simulink model "PubIfDecisionLM_MDL"  (R2020b)
settings: configuration reference "DspaceConfig" (kept outside this file)
PostLoadFcn:
  | if any(exist('dsrtsu_mdlpostloadfcn', 'file') ~= 0), dsrtsu_mdlpostloadfcn('Execute', bdroot); end
InitFcn:
  | , if any(exist('dsmpb_private', 'file') ~= 0), dsmpb_private('dsmpb_mdlclblib', 'Init', bdroot); end,
undefined symbols (not defined in the file or in its folder): OFM_OBJ_FUSIONTYPE_E, OFM_OBJ_MOVINGSTATE_E, OFM_OBJ_ORIENTATION_E, OFM_OBJ_TYPE_E, P_LM_Cyc, P_LM_EMLHistKapRcdBufSize, P_LM_EMLHistTrajBaseDis, P_LM_EMLHistTrajPNum, P_LM_EMLKapCorrMaxThre, P_LM_EMLMinKapThre, P_LM_EMLPathDisDiffThre, P_LM_EMLQuaFiltPar, P_LM_EMLTurnActKapThre, P_LM_EMLValidQuaThre, P_LM_FntPath1Disgap, P_LM_FntPath1MinDis, P_LM_FntPath1Timegap, P_LM_FntPath2Disgap, P_LM_FntPath2MinDis, P_LM_FntPath2Timegap, P_LM_FntPath3Disgap, P_LM_FntPath3MinDis, P_LM_FntPath3Timegap, P_LM_FusBLParFiltP, P_LM_FusEVDifC2Thre, P_LM_FusEVOPath1AllVSLDisThre, P_LM_FusEVOPath1AllVSLLostNumThre, P_LM_FusEVOPath1AllVSLQuaThre, P_LM_FusEVOPath1OTLFacNLC, P_LM_FusOTLQuaThre, P_LM_FusOTLSW, P_LM_FusParC0Index, P_LM_FusParC1Index, P_LM_FusParC2Index, P_LM_FusParC3Index, P_LM_FusVSLQuaThre, P_LM_FusVSLSW, P_LM_FusVSLValidSteerWheerAngThre, P_LM_FusVSLValidVxvThre, P_LM_LaneWidth, P_LM_OTLBufTPInfoEvaFactor, P_LM_OTLObjNum, P_LM_OTLObjSelectAgeThre, P_LM_OTLObjSelectDxAssessVx, P_LM_OTLObjSelectDxThre, P_LM_OTLObjSelectVxThre, P_LM_OTLObjSelectVyAssessDx, P_LM_OTLObjSelectVyThre, P_LM_OTLTrajPntBaseDis, P_LM_OTLTrajStdThre, P_LM_VSLAvailLineNum, P_LM_VSLBLSDiffThre, P_LM_VSLBLSDisRatio, P_LM_VSLFusBLParFiltP_C1, P_LM_VSLFusBLParFiltP_C2, P_LM_VSLFusBLParFiltP_C3, P_LM_VSLFusBLParFiltP_Quality, P_LM_VSLHistTrajBaseDis, P_LM_VSLHistTrajPNum, P_LM_VSLLCC0diff ... (+18)
libraries: simulink x145, LM_LIB x43
(part 2 of 24)

== system PubIfDecisionLM_MDL/Subsystem2/LM_EML/LM_EMLRearPath1 ==
  VxvRef_ms : Inport
  LM_ComEVOffsetX : Inport  Port=2
  LM_ComEVOffsetY : Inport  Port=3
  LM_ComEVOffsetAng : Inport  Port=4
  LM_RearPath1Dis : Inport  Port=5
  LM_RearPath2Dis : Inport  Port=6
  LM_RearPath3Dis : Inport  Port=7
  VehStandstill : Inport  Port=8
  LM_EMLEgoTrajRecorddFlgCalc : Subsystem
  LM_EMLHistTrajCoordinateConvert : Subsystem
  LM_EMLHistTrajRecordBufferInfo : Subsystem
  LM_EMLHistTrajRecordBufferUpdate : Subsystem
  MATLAB Function : MATLAB Function  TreatAsAtomicUnit=on
  Unit Delay1 : UnitDelay  InitialCondition=zeros(80,1)  SampleTime=-1  HasFrameUpgradeWarning=on
  Unit Delay4 : UnitDelay  InitialCondition=zeros(80,1)  SampleTime=-1  HasFrameUpgradeWarning=on
  LM_EMLRearPath1P : Outport
  LM_EMLRearPath1Qulity : Outport  Port=2
  LM_EMLRearPath2P : Outport  Port=3
  LM_EMLRearPath2Qulity : Outport  Port=4
  LM_EMLRearPath3P : Outport  Port=5
  LM_EMLRearPath3Qulity : Outport  Port=6
  wires:
  LM_EMLEgoTrajRecorddFlgCalc/1(LM_EMLHistTrajRcdFlg) -> LM_EMLHistTrajRecordBufferUpdate/3(LM_EMLHistTrajRcdFlg), LM_EMLHistTrajRecordBufferInfo/1(LM_EMLHistTrajRcdFlg)
  LM_EMLHistTrajRecordBufferInfo/1(LM_EMLHistPEndPos) -> LM_EMLHistTrajRecordBufferUpdate/4(LM_EMLHistPEndPos), MATLAB Function/3(LM_EMLHistPEndPos)
  LM_EMLHistTrajCoordinateConvert/1(LM_EMLHistTrajVectXK1Adju) -> LM_EMLHistTrajRecordBufferUpdate/1(LM_EMLHistTrajVectXK1Adju)
  LM_EMLHistTrajRecordBufferUpdate/2(LM_EMLHistTrajVectY) -> Unit Delay4/1, MATLAB Function/2(LM_EMLHistTrajVectY)
  VehStandstill/1 -> LM_EMLEgoTrajRecorddFlgCalc/1(VehStandstill), LM_EMLHistTrajCoordinateConvert/6(VehStandstill)
  LM_ComEVOffsetX/1 -> LM_EMLHistTrajCoordinateConvert/3(LM_ComEVOffsetX)
  LM_ComEVOffsetY/1 -> LM_EMLHistTrajCoordinateConvert/4(LM_ComEVOffsetY)
  VxvRef_ms/1 -> LM_EMLEgoTrajRecorddFlgCalc/2(VxvRef_ms)
  LM_EMLHistTrajCoordinateConvert/2(LM_EMLHistTrajVectYK1Adju) -> LM_EMLHistTrajRecordBufferUpdate/2(LM_EMLHistTrajVectYK1Adju)
  LM_ComEVOffsetAng/1 -> LM_EMLHistTrajCoordinateConvert/5(LM_ComEVOffsetAng)
  LM_EMLHistTrajRecordBufferUpdate/1(LM_EMLHistTrajVectX) -> Unit Delay1/1, MATLAB Function/1(LM_EMLHistTrajVectX)
  LM_EMLHistTrajRecordBufferInfo/2(LM_EMLHistPFristPos) -> MATLAB Function/4(LM_EMLHistPFristPos)
  LM_EMLHistTrajRecordBufferInfo/3(LM_EMLHistPNum) -> MATLAB Function/5(LM_EMLHistPNum)
  MATLAB Function/1(LM_EMLRearPath1P) -> LM_EMLRearPath1P/1  "LM_EMLRearPath1P"
  MATLAB Function/2(LM_EMLRearPath1Qulity) -> LM_EMLRearPath1Qulity/1  "LM_EMLRearPath1Qulity"
  MATLAB Function/6(LM_EMLRearPath3Qulity) -> LM_EMLRearPath3Qulity/1  "LM_EMLRearPath3Qulity"
  MATLAB Function/3(LM_EMLRearPath2P) -> LM_EMLRearPath2P/1  "LM_EMLRearPath2P"
  MATLAB Function/4(LM_EMLRearPath2Qulity) -> LM_EMLRearPath2Qulity/1  "LM_EMLRearPath2Qulity"
  MATLAB Function/5(LM_EMLRearPath3P) -> LM_EMLRearPath3P/1  "LM_EMLRearPath3P"
  Unit Delay1/1 -> LM_EMLHistTrajCoordinateConvert/1(LM_EMLHistTrajVectXK1)
  Unit Delay4/1 -> LM_EMLHistTrajCoordinateConvert/2(LM_EMLHistTrajVectYK1)
  LM_RearPath1Dis/1 -> MATLAB Function/6(LM_RearPath1Dis)
  LM_RearPath2Dis/1 -> MATLAB Function/7(LM_RearPath2Dis)
  LM_RearPath3Dis/1 -> MATLAB Function/8(LM_RearPath3Dis)

== system PubIfDecisionLM_MDL/Subsystem2/LM_Fusion1/LM_FusBaseLineFilt ==
  DIR_BUS : Inport
  LM_C0Info : Inport  Port=2
  LM_FusBLInfo : Inport  Port=3
  Bus Creator : BusCreator  Inputs=4  OutDataTypeStr=Bus: LM_FusC0InfoBus  NonVirtualBus=on
  Bus Creator1 : BusCreator  Inputs=6  OutDataTypeStr=Bus: LM_FusBLInfoBus  NonVirtualBus=on
  Bus Selector : BusSelector  OutputSignals=LM_LLC0,LM_LRC0,LM_RLC0,LM_RRC0
  Bus Selector1 : BusSelector  OutputSignals=DIR_LC2LeValid,DIR_LC2RigValid
  LM_FusBaseLineC0Filt : Subsystem
  LM_FusBaseLineInfoFilt : Subsystem
  Subsystem1 : Subsystem  Commented=on
  LM_FusBLInfoFilt : Outport
  LM_C0InfoFilt : Outport  Port=2
  wires:
  LM_C0Info/1 -> Bus Selector/1
  DIR_BUS/1 -> Bus Selector1/1
  Bus Selector1/1 -> LM_FusBaseLineC0Filt/1(DIR_LC2LeValid)  "<DIR_LC2LeValid>"
  Bus Selector1/2 -> LM_FusBaseLineC0Filt/2(DIR_LC2RigValid)  "<DIR_LC2RigValid>"
  Bus Selector/1 -> LM_FusBaseLineC0Filt/3(LM_LLC0BefFilt)  "<LM_LLC0>"
  Bus Selector/2 -> LM_FusBaseLineC0Filt/4(LM_LRC0BefFilt)  "<LM_LRC0>"
  Bus Selector/3 -> LM_FusBaseLineC0Filt/5(LM_RLC0BefFilt)  "<LM_RLC0>"
  Bus Selector/4 -> LM_FusBaseLineC0Filt/6(LM_RRC0BefFilt)  "<LM_RRC0>"
  LM_FusBaseLineC0Filt/1(LM_LLC0) -> Bus Creator/1
  LM_FusBaseLineC0Filt/2(LM_LRC0) -> Bus Creator/2
  LM_FusBaseLineC0Filt/3(LM_RLC0) -> Bus Creator/3
  LM_FusBaseLineC0Filt/4(LM_RRC0) -> Bus Creator/4
  Bus Creator/1 -> LM_C0InfoFilt/1  "LM_C0InfoFilt"
  LM_FusBaseLineInfoFilt/1(LM_FusBLFntPath1Info) -> Bus Creator1/1
  LM_FusBaseLineInfoFilt/2(LM_FusBLFntPath2Info) -> Bus Creator1/2
  LM_FusBaseLineInfoFilt/3(LM_FusBLFntPath3Info) -> Bus Creator1/3
  LM_FusBaseLineInfoFilt/4(LM_FusBLRearPath1Info) -> Bus Creator1/4
  LM_FusBaseLineInfoFilt/5(LM_FusBLRearPath2Info) -> Bus Creator1/5
  LM_FusBaseLineInfoFilt/6(LM_FusBLRearPath3Info) -> Bus Creator1/6
  LM_FusBLInfo/1 -> LM_FusBaseLineInfoFilt/1(LM_FusBLInfo)
  Bus Creator1/1 -> LM_FusBLInfoFilt/1  "LM_FusBLInfoFilt"

== system PubIfDecisionLM_MDL/Subsystem2/LM_Fusion1/LM_FusBaseLineInfoCalc ==
  LM_FusBLInfo : Inport
  LM_VSL : Inport  Port=2
  LM_EML : Inport  Port=3
  LM_OTL : Inport  Port=4
  LM_REL : Inport  Port=5
  LM_MAL : Inport  Port=6
  Bus Selector : BusSelector  OutputSignals=LM_FusFntPathK
  LM_FusBLFntPath1 : Subsystem  Commented=on
  LM_FusBLFntPath1130 : Subsystem  Commented=on
  LM_FusBLFntPath2 : Subsystem  Commented=on
  LM_FusBLFntPath3 : Subsystem
  LM_FusBLRearPath : Subsystem
  LM_FusBLFntPath1Info : Outport
  LM_FusBLFntPath2Info : Outport  Port=2
  LM_FusBLFntPath3Info : Outport  Port=3
  LM_FusBLRearPath1Info : Outport  Port=4
  LM_FusBLRearPath2Info : Outport  Port=5
  LM_FusBLRearPath3Info : Outport  Port=6
  wires:
  LM_FusBLInfo/1 -> Bus Selector/1
  LM_FusBLRearPath/1(LM_FusBLRearPath1Info) -> LM_FusBLRearPath1Info/1
  LM_FusBLRearPath/2(LM_FusBLRearPath2Info) -> LM_FusBLRearPath2Info/1
  LM_FusBLRearPath/3(LM_FusBLRearPath3Info) -> LM_FusBLRearPath3Info/1
  LM_EML/1 -> LM_FusBLFntPath3/1(LM_EML)
  LM_VSL/1 -> LM_FusBLRearPath/1(LM_VSL), LM_FusBLFntPath3/2(LM_VSL)
  LM_OTL/1 -> LM_FusBLFntPath3/3(LM_OTL)
  Bus Selector/1 -> LM_FusBLFntPath3/6(LM_FusFntPathK)  "<LM_FusFntPathK>"
  LM_REL/1 -> LM_FusBLFntPath3/4(LM_REL)
  LM_MAL/1 -> LM_FusBLFntPath3/5(LM_MAL)
  LM_FusBLFntPath3/1(LM_FusBLFntPath1Info) -> LM_FusBLFntPath1Info/1
  LM_FusBLFntPath3/2(LM_FusBLFntPath2Info) -> LM_FusBLFntPath2Info/1
  LM_FusBLFntPath3/3(LM_FusBLFntPath3Info) -> LM_FusBLFntPath3Info/1

== system PubIfDecisionLM_MDL/Subsystem2/LM_Fusion1/LM_FusLaneModelInfo ==
  LM_FusBLInfoFilt : Inport
  LM_C0InfoFilt : Inport  Port=2
  LM_ComBus : Inport  Port=3
  LM_FusfCamValidInfo : Inport  Port=4
  Bus Selector : BusSelector  OutputSignals=LM_LLC0
  Bus Selector1 : BusSelector  OutputSignals=LM_PathDisBus
  Bus Selector2 : BusSelector  OutputSignals=LM_LRC0
  Bus Selector3 : BusSelector  OutputSignals=LM_RLC0
  Bus Selector4 : BusSelector  OutputSignals=LM_RRC0
  LM_LLInfo : LM_LIB/LM_LineInfo1  SystemSampleTime=-1  VariantActivationTime=update diagram  Latency=0  AutoFrameSizeCalculation=off
  LM_LRInfo : LM_LIB/LM_LineInfo1  SystemSampleTime=-1  VariantActivationTime=update diagram  Latency=0  AutoFrameSizeCalculation=off
      link override LM_Line_Fnt/LM_Path04/Constant1: Value=1
  LM_RLInfo : LM_LIB/LM_LineInfo1  SystemSampleTime=-1  VariantActivationTime=update diagram  Latency=0  AutoFrameSizeCalculation=off
  LM_RRInfo : LM_LIB/LM_LineInfo1  SystemSampleTime=-1  VariantActivationTime=update diagram  Latency=0  AutoFrameSizeCalculation=off
  Signal Conversion{,1..7} (8 alike) : SignalConversion  OverrideOpt=off
  LM_LINE_LL : Outport  BusOutputAsStruct=on
  LM_LINE_LR : Outport  Port=2  BusOutputAsStruct=on
  LM_LINE_RL : Outport  Port=3  BusOutputAsStruct=on
  LM_LINE_RR : Outport  Port=4  BusOutputAsStruct=on
  wires:
  LM_C0InfoFilt/1 -> Bus Selector4/1, Bus Selector3/1, Bus Selector2/1, Bus Selector/1
  Bus Selector1/1 -> LM_LLInfo/3, LM_RRInfo/3, LM_RLInfo/3, LM_LRInfo/3  "<LM_PathDisBus>"
  LM_FusBLInfoFilt/1 -> LM_LLInfo/1, LM_RRInfo/1, LM_RLInfo/1, LM_LRInfo/1
  Bus Selector/1 -> Signal Conversion2/1  "<LM_LLC0>"
  Bus Selector2/1 -> Signal Conversion1/1  "<LM_LRC0>"
  Bus Selector3/1 -> Signal Conversion/1  "<LM_RLC0>"
  Signal Conversion/1 -> LM_RLInfo/2  "LM_LineC0"
  Signal Conversion1/1 -> LM_LRInfo/2  "LM_LineC0"
  Signal Conversion2/1 -> LM_LLInfo/2  "LM_LineC0"
  Bus Selector4/1 -> Signal Conversion3/1  "<LM_RRC0>"
  Signal Conversion3/1 -> LM_RRInfo/2  "LM_LineC0"
  LM_ComBus/1 -> Bus Selector1/1
  LM_RRInfo/1 -> Signal Conversion7/1
  LM_RLInfo/1 -> Signal Conversion6/1
  LM_LRInfo/1 -> Signal Conversion5/1
  LM_LLInfo/1 -> Signal Conversion4/1
  Signal Conversion5/1 -> LM_LINE_LR/1  "LM_LINE_LR"
  Signal Conversion6/1 -> LM_LINE_RL/1  "LM_LINE_RL"
  Signal Conversion7/1 -> LM_LINE_RR/1  "LM_LINE_RR"
  Signal Conversion4/1 -> LM_LINE_LL/1  "LM_LINE_LL"
  LM_FusfCamValidInfo/1 -> LM_LLInfo/4, LM_RRInfo/4, LM_RLInfo/4, LM_LRInfo/4

== system PubIfDecisionLM_MDL/Subsystem2/LM_Fusion1/LM_FusRatioCalc ==
  LM_VSL : Inport
  LM_EML : Inport  Port=2
  LM_OTL1 : Inport  Port=3
  LM_REL : Inport  Port=4
  LM_MAL : Inport  Port=5
  LM_ComBus : Inport  Port=6
  LM_VIE_BUS : Inport  Port=7
  DIR_BUS : Inport  Port=8
  LM_VCAN_CSA : Inport  Port=9
  Bus Selector : BusSelector  OutputSignals=vxvRefMs
  Bus Selector1 : BusSelector  OutputSignals=SteerWheelAng
  Bus Selector2 : BusSelector  OutputSignals=LM_VSLFntPath1Quality
  Bus Selector3 : BusSelector  OutputSignals=LM_OTLFntPath1Qulity,LM_OTLFntPath2Qulity,LM_OTLFntPath3Qulity
  LM_FusionCase : Subsystem
  LM_Fusion_EMLOnly : Subsystem
  LM_Fusion_EO : Subsystem
  LM_Fusion_EV : Subsystem
  LM_Fusion_EVO : Subsystem
  Merge : Merge  Inputs=4
  Merge1 : Merge  Inputs=4
  Switch Case : SwitchCase  CaseConditions={0,1,2,3}  ShowDefaultCase=off
  LM_C0Info : Outport
  LM_FusRatioInfo : Outport  Port=2
  wires:
  Switch Case/3 -> LM_Fusion_EVO/Action
  Switch Case/1 -> LM_Fusion_EMLOnly/Action
  LM_REL/1 -> LM_FusionCase/5(LM_REL)
  LM_FusionCase/1(LM_FusCase) -> Switch Case/1
  Switch Case/2 -> LM_Fusion_EV/Action
  LM_EML/1 -> LM_Fusion_EMLOnly/1(LM_EML), LM_Fusion_EV/2(LM_EML), LM_Fusion_EO/2(LM_EML), LM_Fusion_EVO/2(LM_EML)
  LM_MAL/1 -> LM_FusionCase/6(LM_MAL)
  LM_OTL1/1 -> LM_Fusion_EO/3(LM_OTL), LM_Fusion_EVO/3(LM_OTL), Bus Selector3/1
  Merge/1 -> LM_FusRatioInfo/1  "LM_FusRatioInfo"
  LM_Fusion_EMLOnly/1(LM_FusBLInfo) -> Merge/1
  LM_Fusion_EV/1(LM_FusBLInfo) -> Merge/2
  Bus Selector2/1 -> LM_FusionCase/1(LM_VSLFntPaht1Quality)  "<LM_VSLFntPath1Quality>"
  Bus Selector3/1 -> LM_FusionCase/2(LM_OTLFntPath1Qulity)  "<LM_OTLFntPath1Qulity>"
  LM_ComBus/1 -> LM_Fusion_EO/4(LM_Com), LM_Fusion_EVO/4(LM_Com), LM_Fusion_EV/4(LM_ComBus)
  LM_VSL/1 -> Bus Selector2/1, LM_Fusion_EVO/1(LM_VSL), LM_Fusion_EV/1(LM_VSL)
  LM_Fusion_EVO/1(LM_FusBLInfo) -> Merge/3
  LM_VIE_BUS/1 -> LM_Fusion_EV/3(LM_VIE_BUS), LM_Fusion_EO/5(LM_VIE_BUS), LM_Fusion_EVO/5(LM_VIE_BUS), Bus Selector/1
  Switch Case/4 -> LM_Fusion_EO/Action
  LM_Fusion_EO/1(LM_FusRatioInfo) -> Merge/4
  LM_Fusion_EMLOnly/2(LM_C0Info) -> Merge1/1
  Merge1/1 -> LM_C0Info/1  "LM_C0InfoBefFilt"
  LM_Fusion_EV/2(LM_C0Info) -> Merge1/2
  LM_Fusion_EVO/2(LM_C0Info) -> Merge1/3
  LM_Fusion_EO/2(LM_C0Info) -> Merge1/4
  DIR_BUS/1 -> LM_Fusion_EV/5(DIR_BUS), LM_Fusion_EO/1(DIR_BUS), LM_Fusion_EVO/6(DIR_BUS)
  Bus Selector3/2 -> LM_FusionCase/3(LM_OTLFntPath2Qulity)  "<LM_OTLFntPath2Qulity>"
  Bus Selector3/3 -> LM_FusionCase/4(LM_OTLFntPath3Qulity)  "<LM_OTLFntPath3Qulity>"
  LM_VCAN_CSA/1 -> Bus Selector1/1
  Bus Selector/1 -> LM_FusionCase/7(vxvRefMs)  "<vxvRefMs>"
  Bus Selector1/1 -> LM_FusionCase/8(SteerWheelAng)  "<SteerWheelAng>"

== system PubIfDecisionLM_MDL/Subsystem2/LM_Fusion1/LM_Fus_BLConnectivityCheck ==
  LM_ComBus : Inport
  LM_FusBLInfoFilt : Inport  Port=2
  Bus Creator : BusCreator  Inputs=6  OutDataTypeStr=Bus: LM_FusBLInfoBus  NonVirtualBus=on
  LM_Fus_BLFntPahtConnectivityCheck : Subsystem
  LM_Fus_BLRearPahtConnectivityCheck : Subsystem
  LM_FusBLInfo : Outport
  wires:
  LM_ComBus/1 -> LM_Fus_BLRearPahtConnectivityCheck/1(LM_ComBus), LM_Fus_BLFntPahtConnectivityCheck/1(LM_ComBus)
  LM_FusBLInfoFilt/1 -> LM_Fus_BLRearPahtConnectivityCheck/2(LM_FusBLInfoFilt), LM_Fus_BLFntPahtConnectivityCheck/2(LM_FusBLInfoFilt)
  LM_Fus_BLFntPahtConnectivityCheck/2(LM_FusBLFntPath2Info) -> Bus Creator/2
  LM_Fus_BLFntPahtConnectivityCheck/1(LM_FusBLFntPath1Info) -> Bus Creator/1
  LM_Fus_BLFntPahtConnectivityCheck/3(LM_FusBLFntPath3Info) -> Bus Creator/3
  Bus Creator/1 -> LM_FusBLInfo/1  "LM_FusBLInfoAdju"
  LM_Fus_BLRearPahtConnectivityCheck/1(LM_FusBLFntPath1Info) -> Bus Creator/4
  LM_Fus_BLRearPahtConnectivityCheck/2(LM_FusBLFntPath2Info) -> Bus Creator/5
  LM_Fus_BLRearPahtConnectivityCheck/3(LM_FusBLFntPath3Info) -> Bus Creator/6

== system PubIfDecisionLM_MDL/Subsystem2/LM_Fusion1/LM_FusfCamValidInfoCalc ==
  LM_FusRatioInfo : Inport
  Bus Creator : BusCreator  Inputs=3
  Bus Selector : BusSelector  OutputSignals=LM_FusFntPathK.LM_FusFntPath1VSLK,LM_FusFntPathK.LM_FusFntPath2VSLK,LM_FusFntPathK.LM_FusFntPath3VSLK
  LM_FusfCamValidInfoCalc : Subsystem
  LM_FusfCamValidInfo : Outport
  wires:
  LM_FusRatioInfo/1 -> Bus Selector/1
  Bus Selector/1 -> LM_FusfCamValidInfoCalc/1(LM_FusFntPath1VSLK)  "<LM_FusFntPath1VSLK>"
  Bus Selector/2 -> LM_FusfCamValidInfoCalc/2(LM_FusFntPath2VSLK)  "<LM_FusFntPath2VSLK>"
  Bus Selector/3 -> LM_FusfCamValidInfoCalc/3(LM_FusFntPath3VSLK)  "<LM_FusFntPath3VSLK>"
  LM_FusfCamValidInfoCalc/1(LM_FusFntPath1fCamValid) -> Bus Creator/1
  LM_FusfCamValidInfoCalc/2(LM_FusFntPath2fCamValid) -> Bus Creator/2
  LM_FusfCamValidInfoCalc/3(LM_FusFntPath3fCamValid) -> Bus Creator/3
  Bus Creator/1 -> LM_FusfCamValidInfo/1  "LM_FusfCamValidInfo"

== system PubIfDecisionLM_MDL/Subsystem2/LM_OTL/LM_OTL_MovObjTrajFit ==
  LM_OTLBufTPVectBus : Inport
  LM_OTLBufTPInfoBus : Inport  Port=2
  LM_ComBus : Inport  Port=3
  LM_OTL_BufTPAssess : Subsystem
  LM_OTL_TrajFit : Subsystem
  OTLInfo : Outport
  wires:
  LM_ComBus/1 -> LM_OTL_BufTPAssess/3(LM_ComBus), LM_OTL_TrajFit/3(LM_ComBus)
  LM_OTLBufTPVectBus/1 -> LM_OTL_BufTPAssess/2(LM_OTLBufTPVectBus), LM_OTL_TrajFit/2(LM_OTLBufTPVectBus)
  LM_OTL_BufTPAssess/1(LM_OTL_BufTrajFlg) -> LM_OTL_TrajFit/1(LM_OTL_BufTrajFlg)
  LM_OTLBufTPInfoBus/1 -> LM_OTL_BufTPAssess/1(LM_OTLBufTPInfoBus)
  LM_OTL_TrajFit/1(OTLInfo) -> OTLInfo/1

== system PubIfDecisionLM_MDL/Subsystem2/LM_OTL/LM_OTL_MovObjTrajRecord3 ==
  LM_OTLBufTPVectBusK1 : Inport
  LM_OTLBufTPInfoBusK1 : Inport  Port=2
  LM_VCAN_ESP : Inport  Port=3
  VIE_BUS : Inport  Port=4
  OFM_OBJS : Inport  Port=5  PortDimensions=1  BusOutputAsStruct=on
  LM_ComBus : Inport  Port=6
  Bus Selector : BusSelector  OutputSignals=Object_ID
  Bus Selector1 : BusSelector  OutputSignals=Object_DX,Object_DY
  Bus Selector3 : BusSelector  OutputSignals=vxvRefMs
  Bus Selector4 : BusSelector  OutputSignals=Object_ID
  LM_OTL_BufLostObjTPValidJudge : Subsystem
  LM_OTL_BufRcdObjLostJudge : Subsystem
  LM_OTL_BufTPCC : Subsystem
  LM_OTL_MovObjSelc : Subsystem
  LM_OTL_ObjAlreadyRcdedJudge : Subsystem
  LM_OTL_ObjRcdFlgJudge : Subsystem
  LM_OTL_ObjStoreInfoCalc : Subsystem
  LM_OTLBufTPVectBus : Outport
  LM_OTLBufTPInfoBus : Outport  Port=2
  wires:
  [OFM_OBJS] -> Bus Selector4/1
  Bus Selector4/1 -> LM_OTL_BufRcdObjLostJudge/3(Object_ID)  "<Object_ID>"
  [OFM_OBJS] -> Bus Selector/1
  [LM_OTLBufTPVectAdjuBus] -> LM_OTL_BufLostObjTPValidJudge/3(LM_OTLBufTPVectAdjuBus)
  LM_OTL_BufTPCC/1(LM_OTLBufTPVectAdjuBus) -> [LM_OTLBufTPVectAdjuBus], LM_OTL_ObjStoreInfoCalc/1(LM_OTLBufTPVectAdjuBus)
  VIE_BUS/1 -> Bus Selector3/1
  Bus Selector3/1 -> LM_OTL_MovObjSelc/1(vxvRefMs)  "<vxvRefMs>"
  [LM_OTLBufTPVectAdjuBus] -> LM_OTL_ObjRcdFlgJudge/5(LM_OTLBufTPVectAdjuBus)
  [LM_OTLBufTPInfoBusK1] -> LM_OTL_ObjRcdFlgJudge/6(LM_OTLBufTPInfoBusK1)
  LM_OTL_BufRcdObjLostJudge/1(LM_OTLRcdObjLostFlg_Bus) -> LM_OTL_BufLostObjTPValidJudge/1(LM_OTLRcdObjLostFlg_Bus)
  LM_OTLBufTPInfoBusK1/1 -> [LM_OTLBufTPInfoBusK1], LM_OTL_ObjAlreadyRcdedJudge/2(LM_OTLBufTPInfoBusK1), LM_OTL_BufLostObjTPValidJudge/2(LM_OTLBufTPInfoBusK1), LM_OTL_BufRcdObjLostJudge/2(LM_OTLRcdObjIDVectK1)
  LM_OTL_ObjAlreadyRcdedJudge/2(LM_OTLObjRcdedFlg_Bus) -> LM_OTL_ObjRcdFlgJudge/1(LM_OTLObjRcdedFlg_Bus), LM_OTL_ObjStoreInfoCalc/3(LM_OTLObjRcdedFlg_Bus)
  Bus Selector/1 -> LM_OTL_ObjAlreadyRcdedJudge/1(Object_ID)  "<Object_ID>"
  OFM_OBJS/1 -> [OFM_OBJS], LM_OTL_MovObjSelc/2(OFM_OBJS)
  [OFM_OBJS] -> Bus Selector1/1
  Bus Selector1/1 -> LM_OTL_ObjRcdFlgJudge/2(Object_Dx)  "<Object_DX>"
  LM_OTL_ObjRcdFlgJudge/1(LM_OTLCurObjRcdFlgBus) -> LM_OTL_ObjStoreInfoCalc/4(LM_OTLCurObjRcdFlgBus)
  LM_OTL_BufLostObjTPValidJudge/1(LM_OTLBufLastTPInfoBus) -> LM_OTL_ObjStoreInfoCalc/8(LM_OTLBufLastTPInfoBus)
  LM_OTL_MovObjSelc/1(LM_OTLInterestObjIndexBus) -> LM_OTL_ObjAlreadyRcdedJudge/3(LM_OTLInterestObjIndexBus), LM_OTL_BufRcdObjLostJudge/1(LM_OTLInterestObjIndexVect), LM_OTL_ObjStoreInfoCalc/6(LM_OTLInterestObjIndexBus), LM_OTL_ObjRcdFlgJudge/4(LM_OTLInterestObjIndexBus)
  LM_OTL_ObjAlreadyRcdedJudge/1(LM_OTLCurObjIDBus) -> LM_OTL_ObjStoreInfoCalc/2(LM_OTLCurObjIDBus)
  LM_OTL_ObjRcdFlgJudge/2(LM_OTLCurObjPositonBus) -> LM_OTL_ObjStoreInfoCalc/5(LM_OTLCurObjPositonBus)
  Bus Selector1/2 -> LM_OTL_ObjRcdFlgJudge/3(Object_Dy)  "<Object_DY>"
  LM_OTL_ObjStoreInfoCalc/2(LM_OTLBufTPInfoBus) -> LM_OTLBufTPInfoBus/1
  LM_OTLBufTPVectBusK1/1 -> LM_OTL_BufTPCC/1(LM_OTLBufTPVectBusK1)
  [LM_OTLBufTPInfoBusK1] -> LM_OTL_ObjStoreInfoCalc/7(LM_OTLBufTPInfoBusK1)
  LM_VCAN_ESP/1 -> LM_OTL_BufTPCC/2(LM_VCAN_ESP)
  LM_ComBus/1 -> LM_OTL_BufTPCC/3(LM_ComBus)
  LM_OTL_ObjStoreInfoCalc/1(LM_OTLBufTPVectBus) -> LM_OTLBufTPVectBus/1

== system PubIfDecisionLM_MDL/Subsystem2/LM_SigPrePro1/Subsystem1 ==
  RFM_LINE_L1_k : Inport
  RFM_LINE_R1_k : Inport  Port=2
  RFM_LINE_L2_k : Inport  Port=3
  RFM_LINE_R2_k : Inport  Port=4
  RFM_LINE_L3_k : Inport  Port=5
  RFM_LINE_R3_k : Inport  Port=6
  RFM_LINE_CL_k : Inport  Port=7
  RFM_LINE_LB_k : Inport  Port=8
  RFM_LINE_RB_k : Inport  Port=9
  LM_RFMLineInfoFilter : Subsystem
  Subsystem : Subsystem
  LM_InputLineInfo : Outport
  wires:
  Subsystem/7(RFM_LINE_CL) -> LM_RFMLineInfoFilter/7(RFM_LINE_CL)
  Subsystem/5(RFM_LINE_L3) -> LM_RFMLineInfoFilter/5(RFM_LINE_L3)
  Subsystem/3(RFM_LINE_L2) -> LM_RFMLineInfoFilter/3(RFM_LINE_L2)
  Subsystem/2(RFM_LINE_R1) -> LM_RFMLineInfoFilter/2(RFM_LINE_R1)
  Subsystem/1(RFM_LINE_L1) -> LM_RFMLineInfoFilter/1(RFM_LINE_L1)
  Subsystem/6(RFM_LINE_R3) -> LM_RFMLineInfoFilter/6(RFM_LINE_R3)
  Subsystem/4(RFM_LINE_R2) -> LM_RFMLineInfoFilter/4(RFM_LINE_R2)
  Subsystem/8(RFM_LINE_LB) -> LM_RFMLineInfoFilter/8(RFM_LINE_LB)
  Subsystem/9(RFM_LINE_RB) -> LM_RFMLineInfoFilter/9(RFM_LINE_RB)
  LM_RFMLineInfoFilter/1(LM_InputLineInfo) -> LM_InputLineInfo/1
  RFM_LINE_L1_k/1 -> Subsystem/1(RFM_LINE_L1_k)
  RFM_LINE_R1_k/1 -> Subsystem/2(RFM_LINE_R1_k)
  RFM_LINE_R2_k/1 -> Subsystem/4(RFM_LINE_R2_k)
  RFM_LINE_L3_k/1 -> Subsystem/5(RFM_LINE_L3_k)
  RFM_LINE_L2_k/1 -> Subsystem/3(RFM_LINE_L2_k)
  RFM_LINE_LB_k/1 -> Subsystem/8(RFM_LINE_LB_k)
  RFM_LINE_R3_k/1 -> Subsystem/6(RFM_LINE_R3_k)
  RFM_LINE_CL_k/1 -> Subsystem/7(RFM_LINE_CL_k)
  RFM_LINE_RB_k/1 -> Subsystem/9(RFM_LINE_RB_k)

== system PubIfDecisionLM_MDL/Subsystem2/LM_VSL/LM_VSLFntPath ==
  LM_InputLineInfo : Inport
  LM_ComBus : Inport  Port=2
  LM_InputEHRInfo : Inport  Port=3
  Bus Creator : BusCreator  Inputs=8
  Bus Selector : BusSelector  OutputSignals=LM_LINE_L2.bIsLineExist,LM_LINE_L1.bIsLineExist,LM_LINE_R1.bIsLineExist,LM_LINE_R2.bIsLineExist,LM_LINE_L2.dQuality,LM_LINE_L1.dQuality,LM_LINE_R1.dQuality,LM_LINE_R2.dQuality,LM_LINE_L2.dDisFront,LM_LINE_L1.dDisFront,LM_LINE_R1.dDisFront,LM_LINE_R2.dDisFront,LM_LINE_L2.dDisStart,LM_LINE_L1.dDisStart,LM_LINE_R1.dDisStart,LM_LINE_R2.dDisStart,LM_LINE_L2.dC0V,LM_LINE_L1.dC0V,LM_LINE_R1.dC0V,LM_LINE_R2.dC0V,LM_LINE_L2.dC1V,LM_LINE_L1.dC1V,LM_LINE_R1.dC1V,LM_LINE_R2.dC1V,LM_LINE_L2.dC2V,LM_LINE_L1.dC2V,LM_LINE_R1.dC2V,LM_LINE_R2.dC2V,LM_LINE_L2.dC3V,LM_LINE_L1.dC3V,LM_LINE_R1.dC3V,LM_LINE_R2.dC3V
  Bus Selector1 : BusSelector  OutputSignals=LM_VSLLineExistVect,LM_VSLLineDisFntVect,LM_VSLLineQualityVect,LM_VSLLineC0Vect,LM_VSLLineC1Vect,LM_VSLLineC2Vect,LM_VSLLineC3Vect
  Bus Selector2 : BusSelector  OutputSignals=LM_ComLineLostNum,LM_ComAllLineLost_flg
  Bus Selector3 : BusSelector  OutputSignals=LM_PathDisBus.LM_FntPath1Dis,LM_PathDisBus.LM_FntPath2Dis,LM_PathDisBus.LM_FntPath3Dis
  Bus Selector4 : BusSelector  OutputSignals=LM_VSLLineC0Vect,LM_VSLLineQualityVect,LM_VSLLineExistVect
  Constant : Constant  Value=P_LM_LaneWidth  OutDataTypeStr=single
  LM_VSLC0Calc1 : Stateflow chart  TreatAsAtomicUnit=on
  LM_VSL_FntPathInfo : Subsystem
  LM_VSL_LineInfoEvalutaion : Subsystem
  LM_VSL_LineInfoReorganization : Subsystem
  LM_VSL_LineQualityCalc : Subsystem
  Signal Conversion{,1..7,24..45,54..55} (32 alike) : SignalConversion  OverrideOpt=off
  Terminator : Terminator
  LM_VSLFntPath1P : Outport
  LM_VSLFntPath1Quality : Outport  Port=2
  LM_VSLFntPath2P : Outport  Port=3
  LM_VSLFntPath2Quality : Outport  Port=4
  LM_VSLFntPath3P : Outport  Port=5
  LM_VSLFntPath3Quality : Outport  Port=6
  LM_VSLBaseDis : Outport  Port=7
  LM_VSLLLC0 : Outport  Port=8
  LM_VSLLRC0 : Outport  Port=9
  LM_VSLRLC0 : Outport  Port=10
  LM_VSLRRC0 : Outport  Port=11
  wires:
  Signal Conversion43/1 -> LM_VSL_LineInfoReorganization/30(LM_VSLL1C3)
  Signal Conversion45/1 -> LM_VSL_LineInfoReorganization/32(LM_VSLR2C3)
  Signal Conversion44/1 -> LM_VSL_LineInfoReorganization/31(LM_VSLR1C3)
  Signal Conversion54/1 -> LM_VSL_LineInfoReorganization/25(LM_VSLL2C2)
  Signal Conversion55/1 -> LM_VSL_LineInfoReorganization/26(LM_VSLL1C2)
  Signal Conversion42/1 -> LM_VSL_LineInfoReorganization/29(LM_VSLL2C3)
  Signal Conversion40/1 -> LM_VSL_LineInfoReorganization/27(LM_VSLR1C2)
  Signal Conversion41/1 -> LM_VSL_LineInfoReorganization/28(LM_VSLR2C2)
  Signal Conversion39/1 -> LM_VSL_LineInfoReorganization/10(LM_VSLL1dDisFront)
  Signal Conversion38/1 -> LM_VSL_LineInfoReorganization/9(LM_VSLL2dDisFront)
  Signal Conversion36/1 -> LM_VSL_LineInfoReorganization/17(LM_VSLL2C0)
  Signal Conversion37/1 -> LM_VSL_LineInfoReorganization/18(LM_VSLL1C0)
  Signal Conversion35/1 -> LM_VSL_LineInfoReorganization/24(LM_VSLR2C1)
  Signal Conversion34/1 -> LM_VSL_LineInfoReorganization/23(LM_VSLR1C1)
  Signal Conversion30/1 -> LM_VSL_LineInfoReorganization/19(LM_VSLR1C0)
  Signal Conversion33/1 -> LM_VSL_LineInfoReorganization/22(LM_VSLL1C1)
  Signal Conversion31/1 -> LM_VSL_LineInfoReorganization/20(LM_VSLR2C0)
  Signal Conversion32/1 -> LM_VSL_LineInfoReorganization/21(LM_VSLL2C1)
  Signal Conversion26/1 -> LM_VSL_LineInfoReorganization/13(LM_VSLL2dDisStart)
  Signal Conversion28/1 -> LM_VSL_LineInfoReorganization/15(LM_VSLR1dDisStart)
  Signal Conversion27/1 -> LM_VSL_LineInfoReorganization/14(LM_VSLL1dDisStart)
  Signal Conversion29/1 -> LM_VSL_LineInfoReorganization/16(LM_VSLR2dDisStart)
  Signal Conversion25/1 -> LM_VSL_LineInfoReorganization/12(LM_VSLR2dDisFront)
  Signal Conversion24/1 -> LM_VSL_LineInfoReorganization/11(LM_VSLR1dDisFront)
  Signal Conversion7/1 -> LM_VSL_LineInfoReorganization/8(LM_VSLR2dQuality)
  Signal Conversion6/1 -> LM_VSL_LineInfoReorganization/7(LM_VSLR1dQuality)
  Signal Conversion5/1 -> LM_VSL_LineInfoReorganization/6(LM_VSLL1dQuality)
  Signal Conversion4/1 -> LM_VSL_LineInfoReorganization/5(LM_VSLL2dQuality)
  Signal Conversion3/1 -> LM_VSL_LineInfoReorganization/4(LM_VSLR2bIsLineExist)
  Signal Conversion2/1 -> LM_VSL_LineInfoReorganization/3(LM_VSLR1bIsLineExist)
  Signal Conversion1/1 -> LM_VSL_LineInfoReorganization/2(LM_VSLL1bIsLineExist)
  Signal Conversion/1 -> LM_VSL_LineInfoReorganization/1(LM_VSLL2bIsLineExist)
  LM_VSLC0Calc1/3(LM_VSLRLC0) -> LM_VSLRLC0/1  "LM_VSLRLC0"
  LM_InputEHRInfo/1 -> Terminator/1
  LM_VSLC0Calc1/1(LM_VSLLLC0) -> LM_VSLLLC0/1  "LM_VSLLLC0"
  LM_VSLC0Calc1/2(LM_VSLLRC0) -> LM_VSLLRC0/1  "LM_VSLLRC0"
  LM_VSLC0Calc1/4(LM_VSLRRC0) -> LM_VSLRRC0/1  "LM_VSLRRC0"
  Constant/1 -> LM_VSLC0Calc1/4(P_LM_LaneWidth)
  LM_VSL_LineInfoEvalutaion/4(LM_VSLBaseQuality) -> LM_VSL_LineQualityCalc/1(LM_VSLBaseQuality)
  Bus Selector4/3 -> LM_VSLC0Calc1/3(LM_VSLLineExistVect)  "<LM_VSLLineExistVect>"
  Bus Selector4/1 -> LM_VSLC0Calc1/1(LM_VSLLineC0Vect)  "<LM_VSLLineC0Vect>"
  Bus Selector4/2 -> LM_VSLC0Calc1/2(LM_VSLLineQualityVect)  "<LM_VSLLineQualityVect>"
  Bus Creator/1 -> Bus Selector1/1, Bus Selector4/1
  [LM_ComBus] -> Bus Selector3/1
  LM_VSL_FntPathInfo/2(LM_VSLFntPath2P) -> LM_VSLFntPath2P/1
  LM_VSL_FntPathInfo/3(LM_VSLFntPath3P) -> LM_VSLFntPath3P/1
  LM_VSL_FntPathInfo/1(LM_VSLFntPath1P) -> LM_VSLFntPath1P/1
  Bus Selector3/1 -> LM_VSL_LineQualityCalc/3(LM_FntPath1Dis)  "<LM_FntPath1Dis>"
  Bus Selector3/3 -> LM_VSL_LineQualityCalc/5(LM_FntPath3Dis)  "<LM_FntPath3Dis>"
  Bus Selector3/2 -> LM_VSL_LineQualityCalc/4(LM_FntPath2Dis)  "<LM_FntPath2Dis>"
  LM_VSL_LineQualityCalc/3(LM_VSLFntPath3Quality) -> LM_VSLFntPath3Quality/1  "LM_VSLFntPath3Quality"
  LM_VSL_LineQualityCalc/2(LM_VSLFntPath2Quality) -> LM_VSLFntPath2Quality/1  "LM_VSLFntPath2Quality"
  LM_VSL_LineQualityCalc/1(LM_VSLFntPath1Quality) -> LM_VSLFntPath1Quality/1  "LM_VSLFntPath1Quality"
  Bus Selector1/4 -> LM_VSL_LineInfoEvalutaion/6(LM_VSLLineC0Vect)  "<LM_VSLLineC0Vect>"
  Bus Selector2/2 -> LM_VSL_LineInfoEvalutaion/2(LM_ComAllLineLost_flg)  "<LM_ComAllLineLost_flg>"
  Bus Selector/6 -> Signal Conversion5/1  "<dQuality>"
  Bus Selector1/3 -> LM_VSL_LineInfoEvalutaion/5(LM_VSLLineQualityVect)  "<LM_VSLLineQualityVect>"
  Bus Selector/9 -> Signal Conversion38/1  "<dDisFront>"
  LM_VSL_LineInfoEvalutaion/1(LM_VSLBaseC1) -> LM_VSL_FntPathInfo/1(LM_VSLBaseC1)  "LM_VSLBaseC1"
  Bus Selector/21 -> Signal Conversion32/1  "<dC1V>"
  Bus Selector/32 -> Signal Conversion45/1  "<dC3V>"
  Bus Selector/11 -> Signal Conversion24/1  "<dDisFront>"
  Bus Selector/10 -> Signal Conversion39/1  "<dDisFront>"
  Bus Selector/23 -> Signal Conversion34/1  "<dC1V>"
  Bus Selector/4 -> Signal Conversion3/1  "<bIsLineExist>"
  LM_VSL_LineInfoEvalutaion/2(LM_VSLBaseC2) -> LM_VSL_FntPathInfo/2(LM_VSLBaseC2)  "LM_VSLBaseC2"
  LM_VSL_LineInfoEvalutaion/3(LM_VSLBaseC3) -> LM_VSL_FntPathInfo/3(LM_VSLBaseC3)  "LM_VSLBaseC3"
  Bus Selector/31 -> Signal Conversion44/1  "<dC3V>"
  Bus Selector/3 -> Signal Conversion2/1  "<bIsLineExist>"
  LM_VSL_LineInfoReorganization/4(LM_VSLLineDisStartVect) -> Bus Creator/4
  Bus Selector/18 -> Signal Conversion37/1  "<dC0V>"
  Bus Selector/16 -> Signal Conversion29/1  "<dDisStart>"
  LM_ComBus/1 -> [LM_ComBus], Bus Selector2/1
  Bus Selector/2 -> Signal Conversion1/1  "<bIsLineExist>"
  LM_VSL_LineInfoReorganization/2(LM_VSLLineQualityVect) -> Bus Creator/2
  Bus Selector1/1 -> LM_VSL_LineInfoEvalutaion/3(LM_VSLLineExistVect)  "<LM_VSLLineExistVect>"
  LM_VSL_LineInfoEvalutaion/5(LM_VSLLineMaxDis) -> LM_VSL_LineQualityCalc/2(LM_VSLBaseDis), LM_VSLBaseDis/1  "LM_VSLBaseDis"
  Bus Selector/5 -> Signal Conversion4/1  "<dQuality>"
  Bus Selector1/7 -> LM_VSL_LineInfoEvalutaion/9(LM_VSLLineC3Vect)  "<LM_VSLLineC3Vect>"
  Bus Selector1/6 -> LM_VSL_LineInfoEvalutaion/8(LM_VSLLineC2Vect)  "<LM_VSLLineC2Vect>"
  Bus Selector/30 -> Signal Conversion43/1  "<dC3V>"
  Bus Selector/17 -> Signal Conversion36/1  "<dC0V>"
  LM_VSL_LineInfoReorganization/6(LM_VSLLineC1Vect) -> Bus Creator/6
  Bus Selector/20 -> Signal Conversion31/1  "<dC0V>"
  Bus Selector/24 -> Signal Conversion35/1  "<dC1V>"
  Bus Selector1/2 -> LM_VSL_LineInfoEvalutaion/4(LM_VSLLineDisFntVect)  "<LM_VSLLineDisFntVect>"
  Bus Selector/13 -> Signal Conversion26/1  "<dDisStart>"
  Bus Selector2/1 -> LM_VSL_LineInfoEvalutaion/1(LM_ComLineLostNum)  "<LM_ComLineLostNum>"
  Bus Selector/15 -> Signal Conversion28/1  "<dDisStart>"
  LM_InputLineInfo/1 -> Bus Selector/1
  Bus Selector/19 -> Signal Conversion30/1  "<dC0V>"
  LM_VSL_LineInfoReorganization/3(LM_VSLLineDisFntVect) -> Bus Creator/3
  Bus Selector/12 -> Signal Conversion25/1  "<dDisFront>"
  LM_VSL_LineInfoReorganization/1(LM_VSLLineExistVect) -> Bus Creator/1
  Bus Selector/8 -> Signal Conversion7/1  "<dQuality>"
  Bus Selector/25 -> Signal Conversion54/1  "<dC2V>"
  Bus Selector/26 -> Signal Conversion55/1  "<dC2V>"
  Bus Selector/28 -> Signal Conversion41/1  "<dC2V>"
  Bus Selector/22 -> Signal Conversion33/1  "<dC1V>"
  Bus Selector/29 -> Signal Conversion42/1  "<dC3V>"
  Bus Selector/7 -> Signal Conversion6/1  "<dQuality>"
  LM_VSL_LineInfoReorganization/7(LM_VSLLineC2Vect) -> Bus Creator/7
  Bus Selector/27 -> Signal Conversion40/1  "<dC2V>"
  LM_VSL_LineInfoReorganization/5(LM_VSLLineC0Vect) -> Bus Creator/5
  Bus Selector/1 -> Signal Conversion/1  "<bIsLineExist>"
  Bus Selector/14 -> Signal Conversion27/1  "<dDisStart>"
  LM_VSL_LineInfoReorganization/8(LM_VSLLineC3Vect) -> Bus Creator/8
  Bus Selector1/5 -> LM_VSL_LineInfoEvalutaion/7(LM_VSLLineC1Vect)  "<LM_VSLLineC1Vect>"

== system PubIfDecisionLM_MDL/Subsystem2/LM_VSL/LM_VSLRearPath ==
  LM_VSLFntPath1P : Inport
  LM_ComBus : Inport  Port=2
  RFM_LINE : Inport  Port=3
  VIE_BUS : Inport  Port=4
  LM_VCAN_ESP : Inport  Port=5
  Bus Selector : BusSelector  OutputSignals=vxvRefMs
  Bus Selector1 : BusSelector  OutputSignals=VehStandstill
  Bus Selector2 : BusSelector  OutputSignals=LM_PathDisBus.LM_RearPath1Dis,LM_PathDisBus.LM_RearPath2Dis,LM_PathDisBus.LM_RearPath3Dis
  Bus Selector3 : BusSelector  OutputSignals=signal7.LM_ComEVOffsetX,signal7.LM_ComEVOffsetY,signal7.LM_ComEVOffsetAng
  Constant : Constant  Value=P_LM_VSLRearLaneQualityRatio
  Constant1 : Constant  Value=P_LM_VSLRearLanePolyfitQualityRatio
  LM_VSLC0Calc : Subsystem
  LM_VSLHistLineInfoCoordinateConvert : Subsystem
  LM_VSLHistLineInfoRcdBufferInfo : Subsystem
  LM_VSLHistLineInfoRcdBufferUpdate : Subsystem
  LM_VSLHistLineInfoRcdFlgCalc : Subsystem
  LM_VSLLaChgC0JumpJudge : Subsystem
  MATLAB Function1 : MATLAB Function  TreatAsAtomicUnit=on
  Unit Delay{2..5} (4 alike) : UnitDelay  InitialCondition=zeros(60,1)  SampleTime=-1  HasFrameUpgradeWarning=on
  LM_VSLRearPath1P : Outport
  LM_VSLRearPath1Qulity : Outport  Port=2
  LM_VSLRearPath2P : Outport  Port=3
  LM_VSLRearPath2Qulity : Outport  Port=4
  LM_VSLRearPath3P : Outport  Port=5
  LM_VSLRearPath3Qulity : Outport  Port=6
  wires:
  Constant1/1 -> MATLAB Function1/12(P_LM_VSLRearLanePolyfitQualityRatio)
  Constant/1 -> MATLAB Function1/11(P_LM_VSLRearLaneQualityRatio)
  LM_VSLC0Calc/2(LM_VSLRLC0) -> LM_VSLHistLineInfoRcdBufferUpdate/7(LM_VSLRLC0), LM_VSLLaChgC0JumpJudge/2(LM_VSLRLC0)  "LM_VSL_RearRLC0"
  LM_VSLHistLineInfoRcdFlgCalc/1(LM_VSLHistLineInfoRcdFlg) -> LM_VSLHistLineInfoRcdBufferInfo/1(LM_VSLHistLineInfoRcdFlg), [LM_VSLHistLineInfoRcdFlg]  "LM_VSLHistLineInfoRcdFlg"
  LM_VSLLaChgC0JumpJudge/1(LM_VSLLaChgC0JumpFlg) -> LM_VSLHistLineInfoRcdBufferUpdate/8(LM_VSLLaChgC0JumpFlg)  "LM_VSLLaChgC0JumpFlg"
  LM_VSLHistLineInfoRcdBufferUpdate/3(LM_VSLRLC0HistInfoX) -> MATLAB Function1/3(LM_VSLRLC0HistInfoX), Unit Delay3/1
  LM_VSLHistLineInfoRcdBufferUpdate/1(LM_VSLLRC0HistInfoX) -> MATLAB Function1/1(LM_VSLLRC0HistInfoX), Unit Delay5/1
  LM_VSLHistLineInfoRcdBufferUpdate/4(LM_VSLRLC0HistInfoY) -> MATLAB Function1/4(LM_VSLRLC0HistInfoY), Unit Delay2/1
  LM_VSLHistLineInfoRcdBufferUpdate/2(LM_VSLLRC0HistInfoY) -> MATLAB Function1/2(LM_VSLLRC0HistInfoY), Unit Delay4/1
  VIE_BUS/1 -> Bus Selector/1
  Bus Selector/1 -> LM_VSLHistLineInfoRcdFlgCalc/2(VxvRef_ms)  "<vxvRefMs>"
  LM_VCAN_ESP/1 -> Bus Selector1/1
  Bus Selector3/1 -> LM_VSLHistLineInfoCoordinateConvert/5(LM_EMLOffsetX)  "<LM_ComEVOffsetX>"
  Bus Selector3/2 -> LM_VSLHistLineInfoCoordinateConvert/6(LM_EMLOffsetY)  "<LM_ComEVOffsetY>"
  Bus Selector3/3 -> LM_VSLHistLineInfoCoordinateConvert/7(LM_EMLOffsetAng)  "<LM_ComEVOffsetAng>"
  LM_VSLHistLineInfoCoordinateConvert/4(LM_VSLRLC0HistInfoYK1Adju) -> LM_VSLHistLineInfoRcdBufferUpdate/4(LM_VSLRLC0HistInfoYK1Adju)
  Unit Delay2/1 -> LM_VSLHistLineInfoCoordinateConvert/4(LM_VSLRLC0HistInfoYK1)
  LM_VSLHistLineInfoCoordinateConvert/3(LM_VSLRLC0HistInfoXK1Adju) -> LM_VSLHistLineInfoRcdBufferUpdate/3(LM_VSLRLC0HistInfoXK1Adju)
  Unit Delay3/1 -> LM_VSLHistLineInfoCoordinateConvert/3(LM_VSLRLC0HistInfoXK1)
  Unit Delay4/1 -> LM_VSLHistLineInfoCoordinateConvert/2(LM_VSLLRC0HistInfoYK1)
  Unit Delay5/1 -> LM_VSLHistLineInfoCoordinateConvert/1(LM_VSLLRC0HistInfoXK1)
  LM_VSLHistLineInfoRcdBufferInfo/1(LM_VSLHistPNum) -> MATLAB Function1/5(LM_VSLHistPNum), LM_VSLLaChgC0JumpJudge/4(LM_VSLHistPNum)  "LM_VSLHistPNum"
  LM_VSLHistLineInfoCoordinateConvert/1(LM_VSLLRC0HistInfoXK1Adju) -> LM_VSLHistLineInfoRcdBufferUpdate/1(LM_VSLLRC0HistInfoXK1Adju)
  LM_VSLHistLineInfoCoordinateConvert/2(LM_VSLLRC0HistInfoYK1Adju) -> LM_VSLHistLineInfoRcdBufferUpdate/2(LM_VSLLRC0HistInfoYK1Adju)
  LM_ComBus/1 -> [LM_ComBus], Bus Selector3/1
  Bus Selector2/2 -> MATLAB Function1/9(LM_RearPath2Dis)  "<LM_RearPath2Dis>"
  Bus Selector2/1 -> MATLAB Function1/8(LM_RearPath1Dis)  "<LM_RearPath1Dis>"
  Bus Selector2/3 -> MATLAB Function1/10(LM_RearPath3Dis)  "<LM_RearPath3Dis>"
  MATLAB Function1/1(LM_VSLRearPath1P) -> LM_VSLRearPath1P/1  "LM_VSLRearPath1P"
  MATLAB Function1/2(LM_VSLRearPath1Qulity) -> LM_VSLRearPath1Qulity/1  "LM_VSLRearPath1Qulity"
  MATLAB Function1/3(LM_VSLRearPath2P) -> LM_VSLRearPath2P/1  "LM_VSLRearPath2P"
  MATLAB Function1/4(LM_VSLRearPath2Qulity) -> LM_VSLRearPath2Qulity/1  "LM_VSLRearPath2Qulity"
  MATLAB Function1/5(LM_VSLRearPath3P) -> LM_VSLRearPath3P/1  "LM_VSLRearPath3P"
  MATLAB Function1/6(LM_VSLRearPath3Qulity) -> LM_VSLRearPath3Qulity/1  "LM_VSLRearPath3Qulity"
  LM_VSLHistLineInfoRcdBufferInfo/2(LM_VSLHistPEndPos) -> MATLAB Function1/6(LM_EMLHistPEndPos), LM_VSLHistLineInfoRcdBufferUpdate/9(LM_VSLHistPEndPos)  "LM_VSLHistPEndPos"
  RFM_LINE/1 -> LM_VSLC0Calc/1(RFM_LINE)
  LM_VSLC0Calc/1(LM_VSLLRC0) -> LM_VSLHistLineInfoRcdBufferUpdate/6(LM_VSLLRC0), LM_VSLLaChgC0JumpJudge/1(LM_VSLLRC0)  "LM_VSL_RearLRC0"
  Bus Selector1/1 -> LM_VSLHistLineInfoCoordinateConvert/8(VehStandstill), LM_VSLHistLineInfoRcdFlgCalc/1(VehStandstill)  "<VehStandstill>"
  LM_VSLFntPath1P/1 -> LM_VSLLaChgC0JumpJudge/3(LM_VSLFntPath1P)
  LM_VSLHistLineInfoRcdBufferInfo/3(LM_VSLHistPFristPos) -> MATLAB Function1/7(LM_EMLHistPFristPos)  "LM_VSLHistPFristPos"
  [LM_ComBus] -> Bus Selector2/1
  [LM_VSLHistLineInfoRcdFlg] -> LM_VSLHistLineInfoRcdBufferUpdate/5(LM_VSLHistLineInfoRcdFlg)

== system PubIfDecisionLM_MDL/Subsystem2/DIR/DrivingIntentionRecognition1/DIR_LaneChangeProbCalc ==
  DIR_RightTurnLampOnTime : Inport
  DIR_LeftTurnLampOnTime : Inport  Port=2
  RightTurnSWSts : Inport  Port=3
  LeftTurnSWSts : Inport  Port=4
  SteerWheelAngleSign : Inport  Port=5
  SteerWheelAngle : Inport  Port=6
  vxvRefMs : Inport  Port=7
  LM_LRC0 : Inport  Port=8
  LM_RLC0 : Inport  Port=9
  LM_VSLFntPathBaseC1 : Inport  Port=10
  DIR_EgoVehOnLineJudge : Subsystem
  DIR_LaneChangeLeftProbCalc : Subsystem
  DIR_LaneChangeRightProbCalc : Subsystem
  DIR_LC2LeProb : Outport
  DIR_LC2RigProb : Outport  Port=2
  wires:
  RightTurnSWSts/1 -> DIR_LaneChangeRightProbCalc/8(RightTurnSWSts)
  DIR_RightTurnLampOnTime/1 -> DIR_LaneChangeRightProbCalc/9(DIR_RightTurnLampOnTime)
  LeftTurnSWSts/1 -> DIR_LaneChangeLeftProbCalc/2(LeftTurnSWSts)
  LM_RLC0/1 -> DIR_LaneChangeLeftProbCalc/8(LM_RLC0), DIR_EgoVehOnLineJudge/2(LM_RLC0), DIR_LaneChangeRightProbCalc/2(LM_RLC0)
  LM_LRC0/1 -> DIR_LaneChangeRightProbCalc/3(LM_LRC0), DIR_EgoVehOnLineJudge/1(LM_LRC0), DIR_LaneChangeLeftProbCalc/7(LM_LRC0)
  SteerWheelAngleSign/1 -> DIR_LaneChangeRightProbCalc/6(SteerWheelAngleSign), DIR_LaneChangeLeftProbCalc/4(SteerWheelAngleSign)
  SteerWheelAngle/1 -> DIR_LaneChangeRightProbCalc/7(SteerWheelAngle), DIR_LaneChangeLeftProbCalc/3(SteerWheelAngle)
  DIR_LaneChangeRightProbCalc/1(DIR_LC2RigValid) -> DIR_LC2RigProb/1
  DIR_LaneChangeLeftProbCalc/1(DIR_LC2LeValid) -> DIR_LC2LeProb/1
  DIR_LeftTurnLampOnTime/1 -> DIR_LaneChangeLeftProbCalc/1(DIR_LeftTurnLampOnTime)
  DIR_EgoVehOnLineJudge/1(DIR_EgoVehOnLineValid) -> DIR_LaneChangeLeftProbCalc/9(DIR_EgoVehOnLineValid), DIR_LaneChangeRightProbCalc/1(DIR_EgoVehOnLineValid)
  LM_VSLFntPathBaseC1/1 -> DIR_LaneChangeLeftProbCalc/6(LM_VSLFntPathBaseC1), DIR_LaneChangeRightProbCalc/4(LM_VSLFntPathBaseC1)
  vxvRefMs/1 -> DIR_LaneChangeLeftProbCalc/5(vxvRefMs), DIR_LaneChangeRightProbCalc/5(vxvRefMs)

== system PubIfDecisionLM_MDL/Subsystem2/DIR/DrivingIntentionRecognition1/DIR_TurnDirProbCalc ==
  PsiDtOpt : Inport
  kapTraj : Inport  Port=2
  vxvRefMs : Inport  Port=3
  SteerWheelAngle : Inport  Port=4
  SteerWheelAngleSign : Inport  Port=5
  LeftTurnSWSts : Inport  Port=6
  RightTurnSWSts : Inport  Port=7
  DIR_LeftTurnLampOnTime : Inport  Port=8
  DIR_RightTurnLampOnTime : Inport  Port=9
  DIR_TurnLeftProbCalc : Subsystem
  DIR_TurnRightProbCalc : Subsystem
  DIR_TurnLeftProb : Outport
  DIR_TurnRightProb : Outport  Port=2
  wires:
  PsiDtOpt/1 -> DIR_TurnLeftProbCalc/4(PsiDtOpt), DIR_TurnRightProbCalc/2(PsiDtOpt)
  RightTurnSWSts/1 -> DIR_TurnRightProbCalc/7(RightTurnSWSts)
  DIR_RightTurnLampOnTime/1 -> DIR_TurnRightProbCalc/6(DIR_RightTurnLampOnTime)
  SteerWheelAngleSign/1 -> DIR_TurnLeftProbCalc/7(SteerWheelAngleSign), DIR_TurnRightProbCalc/5(SteerWheelAngleSign)
  SteerWheelAngle/1 -> DIR_TurnLeftProbCalc/6(SteerWheelAngle), DIR_TurnRightProbCalc/4(SteerWheelAngle)
  kapTraj/1 -> DIR_TurnLeftProbCalc/5(kapTraj), DIR_TurnRightProbCalc/3(kapTraj)
  vxvRefMs/1 -> DIR_TurnLeftProbCalc/3(vxvRefMs), DIR_TurnRightProbCalc/1(vxvRefMs)
  LeftTurnSWSts/1 -> DIR_TurnLeftProbCalc/2(LeftTurnSWSts)
  DIR_LeftTurnLampOnTime/1 -> DIR_TurnLeftProbCalc/1(DIR_LeftTurnLampOnTime)
  DIR_TurnRightProbCalc/1(DIR_TurnLeftProb) -> DIR_TurnRightProb/1
  DIR_TurnLeftProbCalc/1(DIR_TurnLeftProb) -> DIR_TurnLeftProb/1

== system PubIfDecisionLM_MDL/Subsystem2/DIR/DrivingIntentionRecognition1/DIR_TurnLampTimeCalc ==
  LeftTurnSWSts : Inport
  RightTurnSWSts : Inport  Port=2
  DIR_LeftTurnLampOnTimeCalc : Subsystem
  DIR_RigTurnLampOnTimeCalc1 : Subsystem
  DIR_LeftTurnLampOnTime : Outport
  DIR_RightTurnLampOnTime : Outport  Port=2
  wires:
  DIR_RigTurnLampOnTimeCalc1/1(DIR_RightTurnLampOnTime) -> DIR_RightTurnLampOnTime/1
  DIR_LeftTurnLampOnTimeCalc/1(DIR_LeftTurnLampOnTime) -> DIR_LeftTurnLampOnTime/1
  RightTurnSWSts/1 -> DIR_RigTurnLampOnTimeCalc1/1(RightTurnSWSts)
  LeftTurnSWSts/1 -> DIR_LeftTurnLampOnTimeCalc/1(LeftTurnSWSts)

== system PubIfDecisionLM_MDL/Subsystem2/LM_ComFcnProcess/LM_DisCalc4EachLine/LM_FrontDisCalc ==
  LM_vxvRefMs : Inport
  Add : Sum
  Add1 : Sum
  Constant : Constant  Commented=on  Value=P_LM_FntPath1Timegap
  Constant1 : Constant  Value=P_LM_FntPath1Disgap
  Constant2 : Constant  Value=P_LM_FntPath1MinDis
  Constant3 : Constant  Value=P_LM_FntPath2Timegap
  Constant4 : Constant  Value=P_LM_FntPath2Disgap
  Constant5 : Constant  Value=P_LM_FntPath2MinDis
  Constant6 : Constant  Value=P_LM_FntPath3Timegap
  Constant7 : Constant  Value=P_LM_FntPath3Disgap
  Constant8 : Constant  Value=P_LM_FntPath3MinDis
  Constant9 : Constant  Value=2.5  OutDataTypeStr=single
  Ground : Ground
  Ground1 : Ground
  Max : MinMax  Function=max  Inputs=2
  Max1 : MinMax  Function=max  Inputs=2
  Max2 : MinMax  Function=max  Inputs=2
  Min : MinMax  Inputs=2
  Min1 : MinMax  Inputs=2
  Min2 : MinMax  Inputs=2
  Product : Product
  Product1 : Product
  Product2 : Product
  LM_FntPath1Dis : Outport
  LM_FntPath2Dis : Outport  Port=2
  LM_FntPath3Dis : Outport  Port=3
  LM_FntPath4Dis : Outport  Port=4
  LM_FntPath5Dis : Outport  Port=5
  wires:
  Constant9/1 -> Product/2
  Ground1/1 -> LM_FntPath5Dis/1  "LM_FntPath5Dis"
  Ground/1 -> LM_FntPath4Dis/1  "LM_FntPath4Dis"
  Min2/1 -> LM_FntPath3Dis/1  "LM_FntPath3Dis"
  Constant8/1 -> Min2/2
  Add1/1 -> Min2/1
  Max2/1 -> Add1/2
  Constant7/1 -> Max2/2
  Product2/1 -> Max2/1
  Constant6/1 -> Product2/2
  Min1/1 -> LM_FntPath2Dis/1, Add1/1  "LM_FntPath2Dis"
  Constant5/1 -> Min1/2
  Add/1 -> Min1/1
  Max1/1 -> Add/2
  Constant4/1 -> Max1/2
  Product1/1 -> Max1/1
  Min/1 -> LM_FntPath1Dis/1, Add/1  "LM_FntPath1Dis"
  Constant2/1 -> Min/2
  Max/1 -> Min/1
  Constant1/1 -> Max/2
  Product/1 -> Max/1
  Constant3/1 -> Product1/2
  LM_vxvRefMs/1 -> Product/1, Product2/1, Product1/1

== system PubIfDecisionLM_MDL/Subsystem2/LM_ComFcnProcess/LM_DisCalc4EachLine/LM_RearDisCalc ==
  Constant : Constant  Value=-30  OutDataTypeStr=single
  Constant1 : Constant  Value=-60  OutDataTypeStr=single
  Constant2 : Constant  Value=-80  OutDataTypeStr=single
  LM_RearPath1Dis : Outport
  LM_RearPath2Dis : Outport  Port=2
  LM_RearPath3Dis : Outport  Port=3
  wires:
  Constant2/1 -> LM_RearPath3Dis/1  "LM_RearPath3Dis"
  Constant1/1 -> LM_RearPath2Dis/1  "LM_RearPath2Dis"
  Constant/1 -> LM_RearPath1Dis/1  "LM_RearPath1Dis"

== system PubIfDecisionLM_MDL/Subsystem2/LM_EML/LM_EMLFntPath1/LM_EMLFntPathParCalc ==
  LM_EMLFntPathkap : Inport
  LM_EMLFntPathPar_C0 : Subsystem
  LM_EMLFntPathPar_C1 : Subsystem
  LM_EMLFntPathPar_C2 : Subsystem
  LM_EMLFntPathPar_C3 : Subsystem
  LM_EML_FntPathPCalc : Subsystem
  LM_EMLFntPath1P : Outport
  LM_EMLFntPath2P : Outport  Port=2
  LM_EMLFntPath3P : Outport  Port=3
  wires:
  LM_EMLFntPathkap/1 -> LM_EMLFntPathPar_C2/1(In1)
  LM_EMLFntPathPar_C0/1(LM_EMLFntPath_C0) -> LM_EML_FntPathPCalc/1(LM_EMLFntPath_C0)
  LM_EMLFntPathPar_C1/1(LM_EMLFntPath_C1) -> LM_EML_FntPathPCalc/2(LM_EMLFntPath_C1)
  LM_EMLFntPathPar_C2/1(LM_EMLFntPath_C2) -> LM_EML_FntPathPCalc/3(LM_EMLFntPath_C2)
  LM_EMLFntPathPar_C3/1(LM_EMLFntPath_C3) -> LM_EML_FntPathPCalc/4(LM_EMLFntPath_C3)
  LM_EML_FntPathPCalc/2(LM_EMLFntPath2P) -> LM_EMLFntPath2P/1
  LM_EML_FntPathPCalc/1(LM_EMLFntPath1P) -> LM_EMLFntPath1P/1
  LM_EML_FntPathPCalc/3(LM_EMLFntPath3P) -> LM_EMLFntPath3P/1

== system PubIfDecisionLM_MDL/Subsystem2/LM_EML/LM_EMLFntPath1/LM_EMLFntPathQualityCalc ==
  VxvRef_ms : Inport
  SteerWheelAngle : Inport  Port=2
  SteerWheelSpd : Inport  Port=3
  1-D Lookup Table : Lookup_n-D  NumberOfTableDimensions=1  BreakpointsForDimension1=single([3,6,10,15,20,35]);  Table=single([0.3499999940395355,0.550000011920929,0.75,0.8999999761581421,0.949999988079071,0.9900000095367432]);  InternalRulePriority=Speed  RndMeth=Simplest  InputSameDT=on
  1-D Lookup Table1 : Lookup_n-D  NumberOfTableDimensions=1  BreakpointsForDimension1=single([0,5,10,15,20,35,50,80,120,170,280]);  Table=single([0.9599999785423279,0.9200000166893005,0.800000011920929,0.699999988079071,0.6000000238418579,0.5,0.30000001192092896,0.3,0.28,0.25,0.2]);  InternalRulePriority=Speed  RndMeth=Simplest  InputSameDT=on
  1-D Lookup Table2 : Lookup_n-D  NumberOfTableDimensions=1  BreakpointsForDimension1=single([5,15,30,50,80,100]);  Table=single([0.9599999785423279,0.800000011920929,0.699999988079071,0.6000000238418579,0.5,0.30000001192092896]);  InternalRulePriority=Speed  RndMeth=Simplest  InputSameDT=on
  1-D Lookup Table3 : Lookup_n-D  NumberOfTableDimensions=1  BreakpointsForDimension1=single([5,10,15,20,30,40]);  Table=single([0,0.25,0.44999998807907104,0.550000011920929,0.6499999761581421,0.8999999761581421]);  InternalRulePriority=Speed  RndMeth=Simplest  InputSameDT=on
  1-D Lookup Table4 : Lookup_n-D  NumberOfTableDimensions=1  BreakpointsForDimension1=single([0,15,20,30,45,50]);  Table=single([0,0,0.35,0.5,0.75,0.8999999761581421]);  InternalRulePriority=Speed  RndMeth=Simplest  InputSameDT=on
  Add : Sum
  Add1 : Sum
  Add2 : Sum
  Constant : Constant  Value=P_LM_EMLQuaFiltPar  OutDataTypeStr=single
  Constant1 : Constant  Value=P_LM_EMLQuaFiltPar  OutDataTypeStr=single
  Constant2 : Constant  Value=P_LM_EMLQuaFiltPar  OutDataTypeStr=single
  Constant3 : Constant  Value=P_LM_EMLValidQuaThre  OutDataTypeStr=single
  Constant4 : Constant  Value=0  OutDataTypeStr=single
  Constant5 : Constant  Value=P_LM_EMLValidQuaThre  OutDataTypeStr=single
  Constant6 : Constant  Value=0  OutDataTypeStr=single
  Product{,1..6} (7 alike) : Product
  Relational Operator : RelationalOperator  Operator=<  OutDataTypeStr=boolean  RndMeth=Simplest
  Relational Operator1 : RelationalOperator  Operator=<  OutDataTypeStr=boolean  RndMeth=Simplest
  Saturation : Saturate  UpperLimit=1  LowerLimit=0.25  OutDataTypeStr=single
  Saturation1 : Saturate  UpperLimit=1  LowerLimit=0  OutDataTypeStr=single
  Saturation2 : Saturate  UpperLimit=1  LowerLimit=0  OutDataTypeStr=single
  Subtract : Sum  Inputs=+-
  Subtract1 : Sum  Inputs=+-
  Subtract2 : Sum  Inputs=+-
  Switch : Switch  Criteria=u2 ~= 0
  Switch1 : Switch  Criteria=u2 ~= 0
  Unit Delay : UnitDelay  SampleTime=-1  HasFrameUpgradeWarning=on
  Unit Delay1 : UnitDelay  SampleTime=-1  HasFrameUpgradeWarning=on
  Unit Delay2 : UnitDelay  SampleTime=-1  HasFrameUpgradeWarning=on
  LM_EMLFntPath1Quality : Outport
  LM_EMLFntPath2Quality : Outport  Port=2
  LM_EMLFntPath3Quality : Outport  Port=3
  wires:
  Saturation1/1 -> Relational Operator1/1, Switch1/3  "LM_EMLFntPath2Quality"
  Add/1 -> Saturation/1
  Subtract1/1 -> Product4/1
  Product4/1 -> Add1/1
  1-D Lookup Table/1 -> Product1/2  "LM_EMLFntPath1QualityFacByVxv"
  1-D Lookup Table4/1 -> Product5/2  "LM_EMLFntPath3QualityFacByVxv"
  Constant/1 -> Product2/2
  Add1/1 -> Saturation1/1  "LM_EMLFntPath2Quality"
  SteerWheelAngle/1 -> 1-D Lookup Table2/1
  1-D Lookup Table3/1 -> Product3/2  "LM_EMLFntPath2QualityFacByVxv"
  Saturation/1 -> Unit Delay/1, LM_EMLFntPath1Quality/1  "LM_EMLFntPath1Quality"
  Product3/1 -> Subtract1/1
  Product5/1 -> Subtract2/1
  Saturation2/1 -> Switch/3, Relational Operator/1
  Unit Delay2/1 -> Add2/2, Subtract2/2
  Subtract2/1 -> Product6/1
  Product6/1 -> Add2/1
  Product2/1 -> Add/1
  Subtract/1 -> Product2/1
  1-D Lookup Table2/1 -> Product/2  "LM_EMLFntPathQualityFacBySteerAng"
  Constant2/1 -> Product6/2
  1-D Lookup Table1/1 -> Product/1  "LM_EMLFntPathBaseQuality"
  Constant1/1 -> Product4/2
  Product/1 -> Product5/1, Product3/1, Product1/1
  VxvRef_ms/1 -> 1-D Lookup Table4/1, 1-D Lookup Table3/1, 1-D Lookup Table/1
  Unit Delay/1 -> Add/2, Subtract/2
  SteerWheelSpd/1 -> 1-D Lookup Table1/1
  Unit Delay1/1 -> Add1/2, Subtract1/2
  Product1/1 -> Subtract/1
  Add2/1 -> Saturation2/1  "LM_EMLFntPath3Quality"
  Constant3/1 -> Relational Operator/2
  Relational Operator/1 -> Switch/2
  Constant4/1 -> Switch/1
  Switch/1 -> Unit Delay2/1, LM_EMLFntPath3Quality/1  "LM_EMLFntPath3Quality"
  Constant6/1 -> Switch1/1
  Relational Operator1/1 -> Switch1/2
  Constant5/1 -> Relational Operator1/2
  Switch1/1 -> Unit Delay1/1, LM_EMLFntPath2Quality/1  "LM_EMLFntPath2Quality"

== system PubIfDecisionLM_MDL/Subsystem2/LM_EML/LM_EMLFntPath1/LM_EMLKapAdjVal ==
  kapTraj : Inport
  DIR_TurnLeftValid : Inport  Port=2
  DIR_TurnRightValid : Inport  Port=3
  Display : Display
  Display1 : Display
  Display2 : Display
  LM_EMLKapAdju : Subsystem
  LM_EMLKapCorrection : Subsystem
  LM_EMLKapValStore : Subsystem
  LM_EMLMinKapWithin3Sec : Subsystem
  LM_EMLKap : Outport
  wires:
  kapTraj/1 -> LM_EMLKapValStore/1(kapTraj), LM_EMLKapCorrection/2(kapTraj), [kapTraj], LM_EMLMinKapWithin3Sec/1(kapTraj)
  LM_EMLKapValStore/1(LM_EMLKapBuf) -> Display/1, LM_EMLMinKapWithin3Sec/2(LM_EMLKapBuf)
  LM_EMLKapValStore/2(LM_EMLKapBufNum) -> LM_EMLMinKapWithin3Sec/3(LM_EMLKapBufNum)
  LM_EMLMinKapWithin3Sec/1(LM_EMLMinKap) -> LM_EMLKapCorrection/1(LM_EMLMinKap)
  DIR_TurnLeftValid/1 -> LM_EMLKapCorrection/3(DIR_TurnLeftValid)
  DIR_TurnRightValid/1 -> LM_EMLKapCorrection/4(DIR_TurnRightValid)
  LM_EMLKapCorrection/1(LM_EMLKapCorr) -> Display1/1, LM_EMLKapAdju/1(LM_EMLKapCorr)
  LM_EMLKapAdju/1(LM_EMLKap) -> Display2/1, LM_EMLKap/1
  [kapTraj] -> LM_EMLKapAdju/2(kapTraj)
